simulink model "problem2d"  (R2022a)
settings: Solver=VariableStepAuto  StartTime=0.0  StopTime=5.0  RelTol=1e-3
settings Model: Creator=prafu  LastModifiedBy=prafu

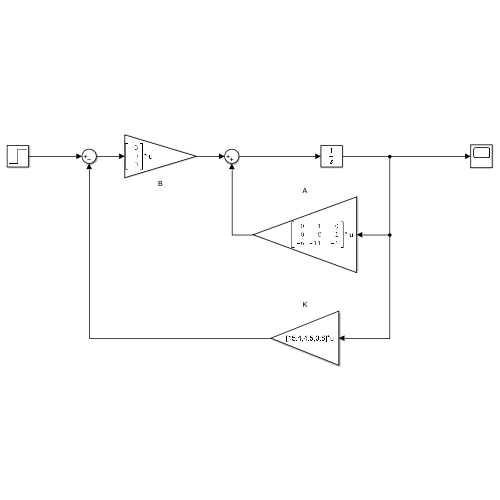
[thumbnail: Simulink's stored preview of the top-level diagram]
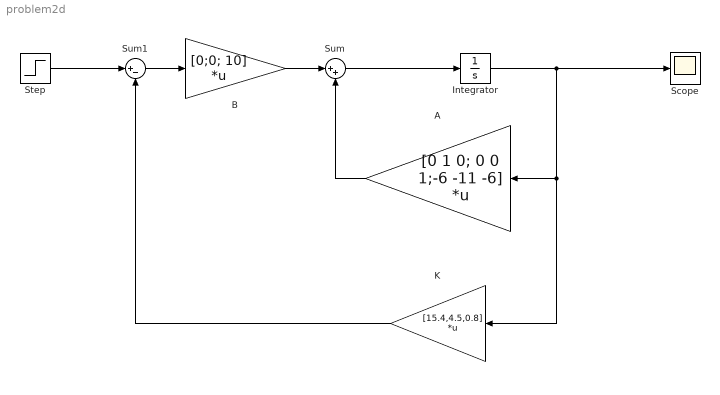
== system problem2d ==
  A : Gain  Gain=[0 1 0; 0 0 1;-6 -11 -6]  Multiplication=Matrix(K*u)
  B : Gain  Gain=[0;0; 10]  Multiplication=Matrix(K*u)
  Integrator : Integrator  InitialCondition=[1;1;1]
  K : Gain  Gain=[15.4,4.5,0.8]  Multiplication=Matrix(K*u)
  Scope : Scope
  Step : Step  SampleTime=0  VectorParams1D=off
  Sum : Sum  Inputs=|++
  Sum1 : Sum  Inputs=|+-
  wires:
  B/1 -> Sum/1
  Sum/1 -> Integrator/1
  Integrator/1 -> K/1, A/1, Scope/1
  A/1 -> Sum/2
  K/1 -> Sum1/2
  Step/1 -> Sum1/1
  Sum1/1 -> B/1
